simulink model "exercise_6_3"  (R2024a)
settings: Solver=VariableStepAuto  StartTime=0.0  StopTime=10.0  RelTol=1e-3  EnableMultiTasking=on
settings Model: Creator=nunkesser  LastModifiedBy=nunkesser
settings SolverCC: AlgebraicLoopSolver=TrustRegion
settings DataIOCC: LimitDataPoints=on  ReturnWorkspaceOutputs=off
settings OptimizationCC: LifeSpan=inf
settings DebuggingCC: UnconnectedInputMsg=warning  UnconnectedOutputMsg=warning  UnconnectedLineMsg=warning  AllowSymbolicDim=off  SFUnexpectedBacktrackingDiag=warning  SFNoUnconditionalDefaultTransitionDiag=warning  SFExecutionAtInitializationDiag=none  ArithmeticOperatorsInVariantConditions=warning
settings ModelReferenceCC: EnableRefExpFcnMdlSchedulingChecks=on  PropagateSignalLabelsOutOfModel=off
settings SFSimCC: SimUseLocalCustomCode=off  CustomCodeUndefinedFunction=UseInterfaceOnly
settings RTWCC: RTWUseLocalCustomCode=off  GPUComputeCapability=3.5
settings CodeAppCC: StateflowObjectComments=on
settings GRTTargetCC: TargetLangStandard=C89/C90 (ANSI)
settings ConfigComp: CovMetricSettings=dw  CovSaveCumulativeToWorkspaceVar=on  CovSaveSingleToWorkspaceVar=on  CovExternalEMLEnable=off

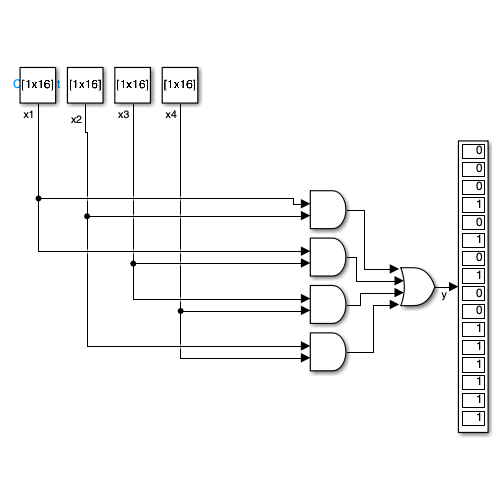
[thumbnail: Simulink's stored preview of the top-level diagram]
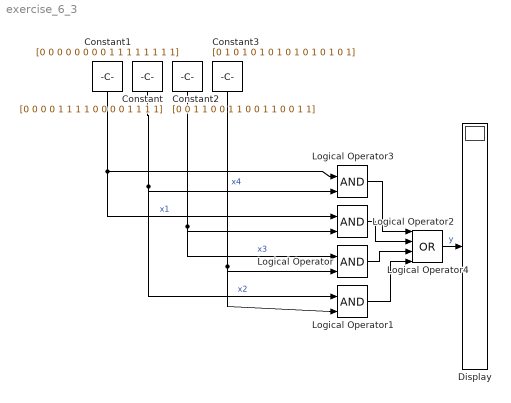
== system exercise_6_3 ==
  Constant : Constant  Value=[0 0 0 0 1 1 1 1 0 0 0 0 1 1 1 1]
  Constant1 : Constant  Value=[0 0 0 0 0 0 0 0 1 1 1 1 1 1 1 1]
  Constant2 : Constant  Value=[0 0 1 1 0 0 1 1 0 0 1 1 0 0 1 1]
  Constant3 : Constant  Value=[0 1 0 1 0 1 0 1 0 1 0 1 0 1 0 1]
  Display : Display
  Logical Operator{,1..3} (4 alike) : Logic  IconShape=distinctive  AllPortsSameDT=off  OutDataTypeStr=boolean
  Logical Operator4 : Logic  Operator=OR  Inputs=4  IconShape=distinctive  AllPortsSameDT=off  OutDataTypeStr=boolean
  wires:
  Logical Operator1/1 -> Logical Operator4/4
  Logical Operator/1 -> Logical Operator4/3
  Logical Operator2/1 -> Logical Operator4/2
  Logical Operator3/1 -> Logical Operator4/1
  Constant3/1 -> Logical Operator/2, Logical Operator1/2  "x4"
  Constant2/1 -> Logical Operator2/2, Logical Operator/1  "x3"
  Constant/1 -> Logical Operator3/2, Logical Operator1/1  "x2"
  Constant1/1 -> Logical Operator3/1, Logical Operator2/1  "x1"
  Logical Operator4/1 -> Display/1  "y"
